simulink model "nmc_full_body_simmechanics_3fbl_2014a"  (R2014a)
settings: Solver=ode23s  StartTime=0.0  StopTime=40  FixedStep=1e-3  MaxStep=ts_max  RelTol=1e-3  AbsTol=1e-4
InitFcn:
  | addpath('../lib');
  | addpath('./init_script');
  | nms_model_MechInit
  | nms_model_ControlInit
undefined symbols (not defined in the file): alphaFmGas, alphaFmGlu, alphaFmHam, alphaFmSol, alphaFmVas, alphaLceHam, alphaLceHfl, alphaLceTa, alphaLceTa1, Amp, amp_var, D12_F, D12_S, D12_T, D13_F, D1G_F, D1G_HAT, D1G_S, D1G_T, freq, freq_var, In_F, In_HAT, In_S, In_T, k_gx, k_gy, k_pressure, m_F, m_HAT, m_S, m_T, mu_slide, mu_stick, sgn, ThPos, v_gx_max, v_gy_max, v_max_pressure, vLimit
libraries: mblibv1 x60, simulink x30, simulink_extras x4, nmc x4
(part 3 of 3)

== system nmc_full_body_simmechanics_3fbl_2014a/Full Body Control (created using the nmc library)/Subsystem/Parameter variation/Amplitude Variation/Up ==
  Amp : Inport
  Enable : EnablePort
  Gain : Gain  Gain=10
  Gain1 : Gain  Gain=0.1
  Ramp : simulink/Sources/Ramp  slope=0.04  start=2  X0=0
  Rounding Function : Rounding  Operator=round
  Saturation : Saturate  UpperLimit=1.5  LowerLimit=0
  Sum : Sum  Inputs=|++
  "AmpUp " : Outport
  wires:
  Ramp/1 -> Gain/1
  Gain/1 -> Rounding Function/1
  Rounding Function/1 -> Gain1/1
  Gain1/1 -> Saturation/1
  Sum/1 -> "AmpUp "/1
  Saturation/1 -> Sum/1
  Amp/1 -> Sum/2

== system nmc_full_body_simmechanics_3fbl_2014a/Full Body Control (created using the nmc library)/Subsystem/Parameter variation/Freq variation/Down ==
  "freq " : Inport
  Enable : EnablePort
  Gain : Gain  Gain=10
  Gain1 : Gain  Gain=0.1
  Ramp : simulink/Sources/Ramp  slope=0.04  start=2  X0=0
  Rounding Function : Rounding  Operator=round
  Saturation : Saturate  UpperLimit=1.5  LowerLimit=0
  Subtract : Sum  Inputs=+-
  "freqDown " : Outport
  wires:
  Saturation/1 -> Subtract/2
  Ramp/1 -> Gain/1
  "freq "/1 -> Subtract/1
  Gain/1 -> Rounding Function/1
  Rounding Function/1 -> Gain1/1
  Gain1/1 -> Saturation/1
  Subtract/1 -> "freqDown "/1

== system nmc_full_body_simmechanics_3fbl_2014a/Full Body Control (created using the nmc library)/Subsystem/Parameter variation/Freq variation/Off  ==
  freq : Inport
  Enable : EnablePort
  "Amp " : Outport
  wires:
  freq/1 -> "Amp "/1

== system nmc_full_body_simmechanics_3fbl_2014a/Full Body Control (created using the nmc library)/Subsystem/Parameter variation/Freq variation/Up ==
  "freq " : Inport
  Enable : EnablePort
  Gain : Gain  Gain=10
  Gain1 : Gain  Gain=0.1
  Ramp : simulink/Sources/Ramp  slope=0.04  start=2  X0=0
  Rounding Function : Rounding  Operator=round
  Saturation : Saturate  UpperLimit=1.5  LowerLimit=0
  Sum : Sum  Inputs=|++
  "freqUp " : Outport
  wires:
  Ramp/1 -> Gain/1
  Gain/1 -> Rounding Function/1
  Rounding Function/1 -> Gain1/1
  Gain1/1 -> Saturation/1
  Sum/1 -> "freqUp "/1
  Saturation/1 -> Sum/1
  "freq "/1 -> Sum/2
